simulink model "test_sim"  (R2024b)
settings: Solver=VariableStepAuto  StartTime=0.0  StopTime=10.0  RelTol=1e-3
undefined symbols (not defined in the file): ctrl, Fw, im, incenc, Lm, Lr, Ls, p, par, Rr
libraries: simulink x2
settings Model: Creator=overflow  LastModifiedBy=overflow

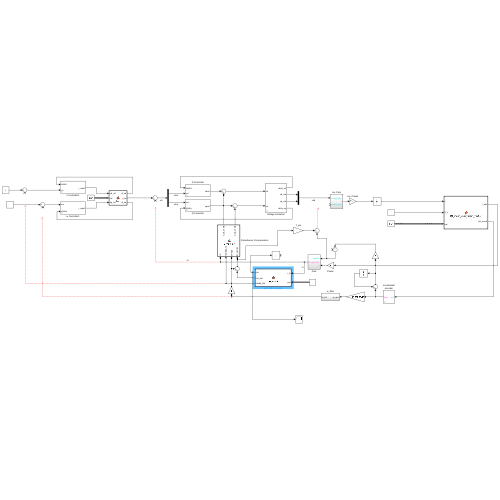
[thumbnail: Simulink's stored preview of the top-level diagram]
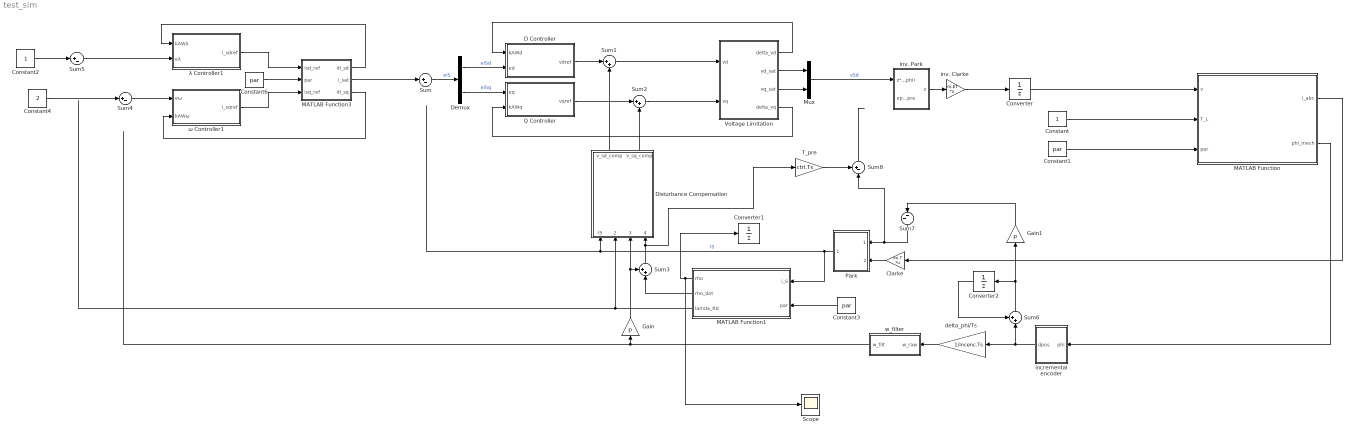
== system test_sim ==
  Clarke : Gain  Gain=im.T  Multiplication=Matrix(K*u)
  Constant : Constant
  Constant1 : Constant  Value=par  OutDataTypeStr=Bus: slBus1
  Constant2 : Constant
  Constant3 : Constant  Value=par  OutDataTypeStr=Bus: slBus1
  Constant4 : Constant  Value=2
  Constant6 : Constant  Value=par  OutDataTypeStr=Bus: slBus1
  Converter : UnitDelay  SampleTime=-1  HasFrameUpgradeWarning=on
  Converter1 : UnitDelay  SampleTime=-1  HasFrameUpgradeWarning=on
  Converter2 : UnitDelay  SampleTime=-1  HasFrameUpgradeWarning=on
  D Controller : Subsystem  mask{Ts=ctrl.Ts, ctrl=ctrl.i}
      mask prompts: Ts "Sampling Time"; ctrl "Controller Struct"
  Demux : Demux  Outputs=2
  Disturbance Compensation : MATLAB Function  TreatAsAtomicUnit=on
  Gain : Gain  Gain=p
  Gain1 : Gain  Gain=p
  MATLAB Function : MATLAB Function  TreatAsAtomicUnit=on
  MATLAB Function1 : MATLAB Function  TreatAsAtomicUnit=on
  MATLAB Function3 : MATLAB Function  TreatAsAtomicUnit=on
  Mux : Mux  Inputs=2
  Park : Subsystem
  Q Controller : Subsystem  mask{Ts=ctrl.Ts, ctrl=ctrl.i}
      mask prompts: Ts "Sampling Time"; ctrl "Controller Struct"
  Scope : Scope
  Sum : Sum  Inputs=|+-
  Sum1 : Sum  Inputs=|++  OutDataTypeStr=double  AccumDataTypeStr=double
  Sum2 : Sum  Inputs=|++  OutDataTypeStr=double  AccumDataTypeStr=double
  Sum3 : Sum  Inputs=++|
  Sum4 : Sum  Inputs=|+-
  Sum5 : Sum  Inputs=|+-
  Sum6 : Sum  Inputs=++|
  Sum7 : Sum  Inputs=--|
  Sum8 : Sum  Inputs=+-|
  T_pre : Gain  Gain=ctrl.Ts  SaturateOnIntegerOverflow=on  OutDataTypeStr=Inherit: Same as input  ParamDataTypeStr=Inherit: Same as input
  Voltage Limitation : Subsystem  mask{Vmax=im.vDC}
      mask prompts: Vmax "Max Voltage"
  delta_phi/Ts : Gain  Gain=1/incenc.Ts  SaturateOnIntegerOverflow=on  OutDataTypeStr=Inherit: Same as input  ParamDataTypeStr=Inherit: Same as input
  incremental encoder : Subsystem  mask{incenc=incenc}
      mask prompts: incenc "Parameterstruct"
  inv. Clarke : Gain  Gain=im.ET  Multiplication=Matrix(K*u)
  inv. Park : Subsystem
  w_filter : Subsystem
  λ Controller1 : Subsystem  mask{Ts=ctrl.Ts, ctrl=ctrl.w}
      mask prompts: Ts "Sampling Time"; ctrl "Controller Struct"
  ω Controller1 : Subsystem  mask{Ts=ctrl.Ts, ctrl=ctrl.w}
      mask prompts: Ts "Sampling Time"; ctrl "Controller Struct"
  wires:
  Demux/1 -> D Controller/2(ed)  "eiSd"
  w_filter/1(w_filt) -> Gain/1
  Sum1/1 -> Voltage Limitation/1(vd)
  Sum3/1 -> T_pre/1, Disturbance Compensation/4(dt_epsilon)
  Disturbance Compensation/1(v_sd_comp) -> Sum1/2
  Voltage Limitation/1(delta_vd) -> D Controller/1(kAWd)
  incremental encoder/1(dpos) -> Sum6/2, delta_phi/Ts/1
  Voltage Limitation/2(vd_sat) -> Mux/1
  T_pre/1 -> Sum8/1
  Voltage Limitation/4(delta_vq) -> Q Controller/2(kAWq)
  MATLAB Function/1(i_abc) -> Clarke/1
  ω Controller1/1(i_sqref) -> MATLAB Function3/3(isq_ref)
  Gain1/1 -> Sum7/2
  Constant/1 -> MATLAB Function/2(T_L)
  Sum4/1 -> ω Controller1/1(eω)
  Sum2/1 -> Voltage Limitation/2("vq ")
  Park/1(z*exp(j*phi)) -> MATLAB Function1/1(i_S), Disturbance Compensation/1(iS)  "iS"
  MATLAB Function1/1(rho) -> Scope/1, Converter1/1
  MATLAB Function1/2(rho_dot) -> Sum3/2
  Sum5/1 -> λ Controller1/2(eλ)
  Constant3/1 -> MATLAB Function1/2(par)
  MATLAB Function3/2(i_sat) -> Sum/1
  MATLAB Function3/1(di_sd) -> λ Controller1/1(kAWλ)
  MATLAB Function/2(phi_mech) -> incremental encoder/1(phi)
  inv. Clarke/1 -> Converter/1
  Constant6/1 -> MATLAB Function3/2(par)
  Demux/2 -> Q Controller/1(eq)  "eiSq"
  Sum8/1 -> ?
  MATLAB Function3/3(di_sq) -> ω Controller1/2(kAWω)
  Clarke/1 -> Park/2(z)
  Converter2/1 -> Sum6/1
  λ Controller1/1(i_sdref) -> MATLAB Function3/1(isd_ref)
  Constant1/1 -> MATLAB Function/3(par)
  MATLAB Function1/3(lamda_Rd) -> Disturbance Compensation/2(lambda_rd)
  Sum7/1 -> Sum8/2, Park/1(-epsilon)
  Sum/1 -> Demux/1  "eiS"
  Converter/1 -> MATLAB Function/1(v)
  Mux/1 -> inv. Park/1(z*exp(j*phi))  "vSd"
  Disturbance Compensation/2(v_sq_comp) -> Sum2/2
  Q Controller/1(vqref) -> Sum2/1
  inv. Park/1(z) -> inv. Clarke/1
  Gain/1 -> Sum3/1, Disturbance Compensation/3(omega)
  D Controller/1(vdref) -> Sum1/1
  Sum6/1 -> Gain1/1, Converter2/1
  Voltage Limitation/3(vq_sat) -> Mux/2
  Constant2/1 -> Sum5/1
  Constant4/1 -> Sum4/1
  delta_phi/Ts/1 -> w_filter/1(w_raw)

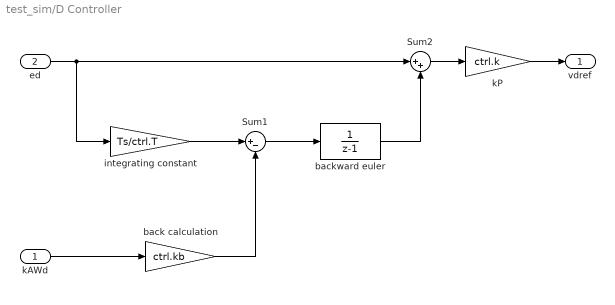
== system test_sim/D Controller ==
  kAWd : Inport
  ed : Inport  Port=2
  Sum1 : Sum  Inputs=|+-
  Sum2 : Sum  Inputs=|++
  back calculation : Gain  Gain=ctrl.kb
  backward euler : DiscreteTransferFcn  Denominator=[1 -1]
  integrating constant : Gain  Gain=Ts/ctrl.T
  kP : Gain  Gain=ctrl.k
  vdref : Outport
  wires:
  Sum1/1 -> backward euler/1
  integrating constant/1 -> Sum1/1
  back calculation/1 -> Sum1/2
  ed/1 -> integrating constant/1, Sum2/1
  Sum2/1 -> kP/1
  kP/1 -> vdref/1
  backward euler/1 -> Sum2/2
  kAWd/1 -> back calculation/1

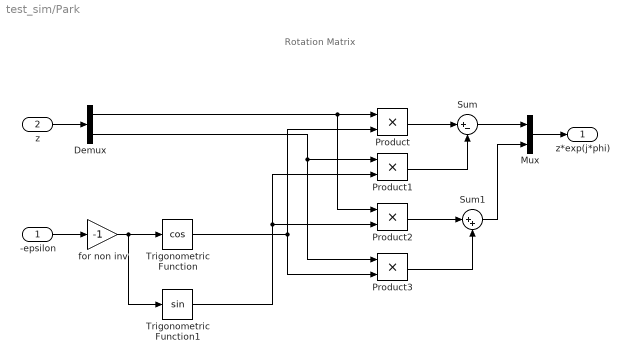
== system test_sim/Park ==
  note: Rotation Matrix
  -epsilon : Inport
  z : Inport  Port=2
  Demux : Demux  Outputs=2
      settings: DisplayOption=none
  Mux : Mux  Inputs=2
  Product{,1..3} (4 alike) : Product  SaturateOnIntegerOverflow=on  OutDataTypeStr=Inherit: Same as first input
  Sum : Sum  Inputs=|+-  SaturateOnIntegerOverflow=on
  Sum1 : Sum  Inputs=|++  SaturateOnIntegerOverflow=on
  Trigonometric Function : Trigonometry  Operator=cos
  Trigonometric Function1 : Trigonometry
  for non inv : Gain  Gain=-1
  z*exp(j*phi) : Outport  PortDimensions=2  VectorParamsAs1DForOutWhenUnconnected=off
  wires:
  Mux/1 -> z*exp(j*phi)/1
  Sum1/1 -> Mux/2
  Sum/1 -> Mux/1
  Product3/1 -> Sum1/2
  Product2/1 -> Sum1/1
  Product1/1 -> Sum/2
  Product/1 -> Sum/1
  Trigonometric Function1/1 -> Product2/2, Product1/2
  Trigonometric Function/1 -> Product3/2, Product/2
  Demux/2 -> Product3/1, Product1/1
  Demux/1 -> Product2/1, Product/1
  z/1 -> Demux/1
  -epsilon/1 -> for non inv/1
  for non inv/1 -> Trigonometric Function1/1, Trigonometric Function/1

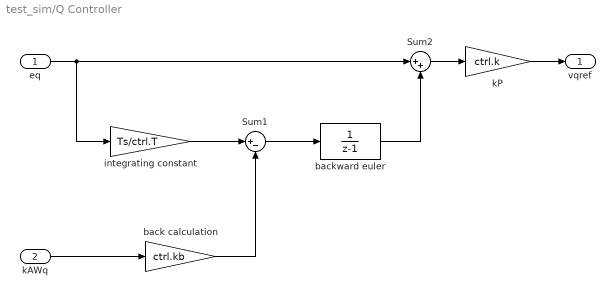
== system test_sim/Q Controller ==
  eq : Inport
  kAWq : Inport  Port=2
  Sum1 : Sum  Inputs=|+-
  Sum2 : Sum  Inputs=|++
  back calculation : Gain  Gain=ctrl.kb
  backward euler : DiscreteTransferFcn  Denominator=[1 -1]
  integrating constant : Gain  Gain=Ts/ctrl.T
  kP : Gain  Gain=ctrl.k
  vqref : Outport
  wires:
  Sum1/1 -> backward euler/1
  integrating constant/1 -> Sum1/1
  back calculation/1 -> Sum1/2
  eq/1 -> integrating constant/1, Sum2/1
  Sum2/1 -> kP/1
  kP/1 -> vqref/1
  backward euler/1 -> Sum2/2
  kAWq/1 -> back calculation/1

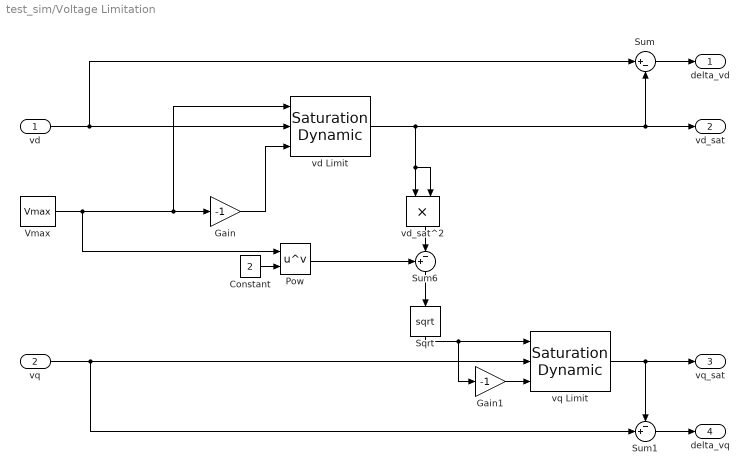
== system test_sim/Voltage Limitation ==
  vd : Inport
  "vq " : Inport  Port=2
  Constant : Constant  Value=2
  Gain : Gain  Gain=-1
  Gain1 : Gain  Gain=-1
  Pow : Math  Operator=pow  RndMeth=Zero
  Sqrt : Sqrt
  Sum : Sum  Inputs=|+-
  Sum1 : Sum  Inputs=-+|
  Sum6 : Sum  Inputs=+-|
  Vmax : Constant  Value=Vmax
  vd Limit : simulink/Discontinuities/Saturation Dynamic  OutMin=[]  OutMax=[]  OutDataTypeStr=Inherit: Same as second input  OutDataType=fixdt(1, 16)  OutScaling=2^-10  DoSatur=off
  vd_sat^2 : Product
  vq Limit : simulink/Discontinuities/Saturation Dynamic  OutMin=[]  OutMax=[]  OutDataTypeStr=Inherit: Same as second input  OutDataType=fixdt(1, 16)  OutScaling=2^-10  DoSatur=off
  delta_vd : Outport  VectorParamsAs1DForOutWhenUnconnected=off
  vd_sat : Outport  Port=2  VectorParamsAs1DForOutWhenUnconnected=off
  vq_sat : Outport  Port=3  VectorParamsAs1DForOutWhenUnconnected=off
  delta_vq : Outport  Port=4  VectorParamsAs1DForOutWhenUnconnected=off
  wires:
  Gain/1 -> vd Limit/3
  vd Limit/1 -> Sum/2, vd_sat/1, vd_sat^2/2, vd_sat^2/1
  Sqrt/1 -> Gain1/1, vq Limit/1
  vq Limit/1 -> Sum1/1, vq_sat/1
  Pow/1 -> Sum6/1
  vd/1 -> Sum/1, vd Limit/2
  Sum6/1 -> Sqrt/1
  "vq "/1 -> vq Limit/2, Sum1/2
  vd_sat^2/1 -> Sum6/2
  Vmax/1 -> Pow/1, Gain/1, vd Limit/1
  Gain1/1 -> vq Limit/3
  Sum/1 -> delta_vd/1
  Sum1/1 -> delta_vq/1
  Constant/1 -> Pow/2

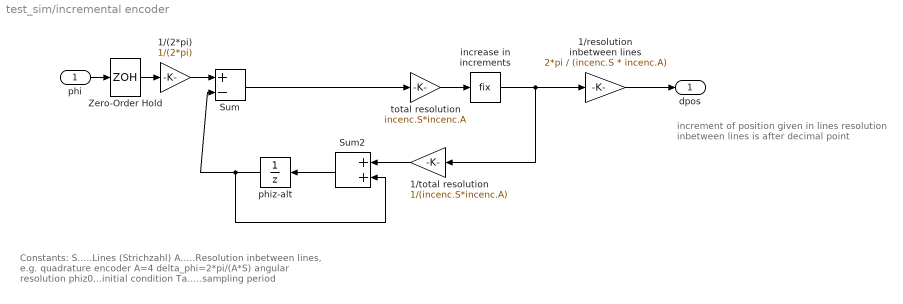
== system test_sim/incremental encoder ==
  note: increment of position given in lines
      | resolution inbetween lines is after decimal point
  note: Constants:
      | S.....Lines (Strichzahl)
      | A.....Resolution inbetween lines, e.g. quadrature encoder A=4
      |        delta_phi=2*pi/(A*S) angular resolution
      | phiz0...initial condition
      | Ta.....sampling period
  phi : Inport
  1/(2*pi) : Gain  Gain=1/(2*pi)  OutDataTypeStr=Inherit: Same as input  ParamDataTypeStr=Inherit: Same as input
  1/resolution inbetween lines : Gain  Gain=2*pi / (incenc.S * incenc.A)  OutDataTypeStr=Inherit: Same as input  ParamDataTypeStr=Inherit: Same as input
  1/total resolution : Gain  Gain=1/(incenc.S*incenc.A)  OutDataTypeStr=Inherit: Same as input  ParamDataTypeStr=Inherit: Same as input
  Sum : Sum  Inputs=+-  InputSameDT=on  OutDataTypeStr=Inherit: Same as first input
  Sum2 : Sum  InputSameDT=on  OutDataTypeStr=Inherit: Same as first input
  Zero-Order Hold : ZeroOrderHold  SampleTime=incenc.Ts
  increase in increments : Rounding  Operator=fix
  phiz-alt : UnitDelay  InitialCondition=incenc.phiz0  SampleTime=incenc.Ts  HasFrameUpgradeWarning=on
  total resolution : Gain  Gain=incenc.S*incenc.A  OutDataTypeStr=Inherit: Same as input  ParamDataTypeStr=Inherit: Same as input
  dpos : Outport  VectorParamsAs1DForOutWhenUnconnected=off
  wires:
  Sum2/1 -> phiz-alt/1
  1/total resolution/1 -> Sum2/1
  1/(2*pi)/1 -> Sum/1
  increase in increments/1 -> 1/resolution inbetween lines/1, 1/total resolution/1
  phi/1 -> Zero-Order Hold/1
  phiz-alt/1 -> Sum2/2, Sum/2
  total resolution/1 -> increase in increments/1
  Sum/1 -> total resolution/1
  Zero-Order Hold/1 -> 1/(2*pi)/1
  1/resolution inbetween lines/1 -> dpos/1

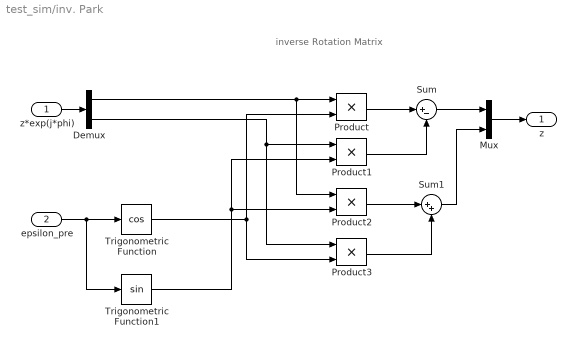
== system test_sim/inv. Park ==
  note: inverse Rotation Matrix
  z*exp(j*phi) : Inport
  epsilon_pre : Inport  Port=2
  Demux : Demux  Outputs=2
      settings: DisplayOption=none
  Mux : Mux  Inputs=2
  Product{,1..3} (4 alike) : Product  SaturateOnIntegerOverflow=on  OutDataTypeStr=Inherit: Same as first input
  Sum : Sum  Inputs=|+-  SaturateOnIntegerOverflow=on
  Sum1 : Sum  Inputs=|++  SaturateOnIntegerOverflow=on
  Trigonometric Function : Trigonometry  Operator=cos
  Trigonometric Function1 : Trigonometry
  z : Outport  PortDimensions=2  VectorParamsAs1DForOutWhenUnconnected=off
  wires:
  z*exp(j*phi)/1 -> Demux/1
  Demux/1 -> Product/1, Product2/1
  epsilon_pre/1 -> Trigonometric Function1/1, Trigonometric Function/1
  Demux/2 -> Product1/1, Product3/1
  Trigonometric Function/1 -> Product/2, Product3/2
  Trigonometric Function1/1 -> Product1/2, Product2/2
  Product/1 -> Sum/1
  Product1/1 -> Sum/2
  Product2/1 -> Sum1/1
  Product3/1 -> Sum1/2
  Sum/1 -> Mux/1
  Sum1/1 -> Mux/2
  Mux/1 -> z/1

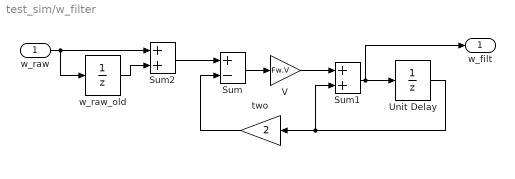
== system test_sim/w_filter ==
  w_raw : Inport
  Sum : Sum  Inputs=+-  SaturateOnIntegerOverflow=on
  Sum1 : Sum  SaturateOnIntegerOverflow=on
  Sum2 : Sum  SaturateOnIntegerOverflow=on
  Unit Delay : UnitDelay  InitialCondition=Fw.w0  SampleTime=Fw.Ts  HasFrameUpgradeWarning=on
  V : Gain  Gain=Fw.V  SaturateOnIntegerOverflow=on  OutDataTypeStr=Inherit: Same as input  ParamDataTypeStr=Inherit: Same as input
  two : Gain  Gain=2  SaturateOnIntegerOverflow=on  OutDataTypeStr=Inherit: Same as input  ParamDataTypeStr=Inherit: Same as input
  w_raw_old : UnitDelay  InitialCondition=Fw.w0  SampleTime=Fw.Ts  HasFrameUpgradeWarning=on
  w_filt : Outport  VectorParamsAs1DForOutWhenUnconnected=off
  wires:
  Sum1/1 -> Unit Delay/1, w_filt/1
  Sum/1 -> V/1
  Sum2/1 -> Sum/1
  V/1 -> Sum1/1
  two/1 -> Sum/2
  Unit Delay/1 -> two/1, Sum1/2
  w_raw_old/1 -> Sum2/2
  w_raw/1 -> w_raw_old/1, Sum2/1

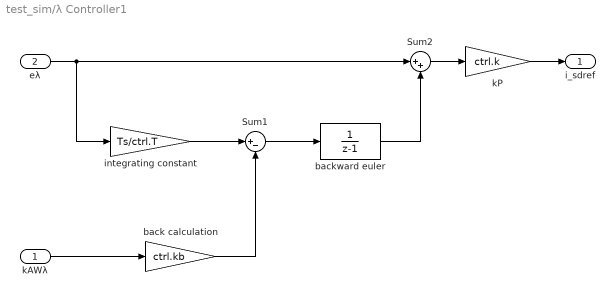
== system test_sim/λ Controller1 ==
  kAWλ : Inport
  eλ : Inport  Port=2
  Sum1 : Sum  Inputs=|+-
  Sum2 : Sum  Inputs=|++
  back calculation : Gain  Gain=ctrl.kb
  backward euler : DiscreteTransferFcn  Denominator=[1 -1]
  integrating constant : Gain  Gain=Ts/ctrl.T
  kP : Gain  Gain=ctrl.k
  i_sdref : Outport
  wires:
  Sum1/1 -> backward euler/1
  integrating constant/1 -> Sum1/1
  back calculation/1 -> Sum1/2
  eλ/1 -> integrating constant/1, Sum2/1
  Sum2/1 -> kP/1
  kP/1 -> i_sdref/1
  backward euler/1 -> Sum2/2
  kAWλ/1 -> back calculation/1

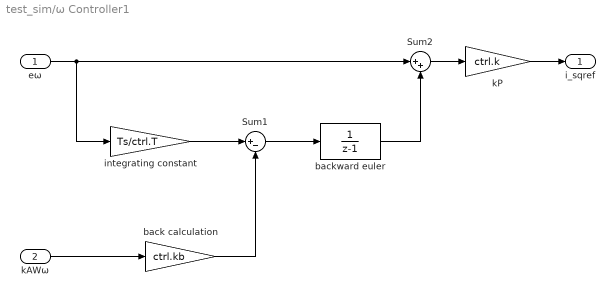
== system test_sim/ω Controller1 ==
  eω : Inport
  kAWω : Inport  Port=2
  Sum1 : Sum  Inputs=|+-
  Sum2 : Sum  Inputs=|++
  back calculation : Gain  Gain=ctrl.kb
  backward euler : DiscreteTransferFcn  Denominator=[1 -1]
  integrating constant : Gain  Gain=Ts/ctrl.T
  kP : Gain  Gain=ctrl.k
  i_sqref : Outport
  wires:
  Sum1/1 -> backward euler/1
  integrating constant/1 -> Sum1/1
  back calculation/1 -> Sum1/2
  eω/1 -> integrating constant/1, Sum2/1
  Sum2/1 -> kP/1
  kP/1 -> i_sqref/1
  backward euler/1 -> Sum2/2
  kAWω/1 -> back calculation/1

== matlab function test_sim/MATLAB Function1 ==
  data: rho output; rho_dot output; i_S input; lamda_Rd output; par input
function [rho, rho_dot, lamda_Rd] = flux_model(i_S, par)

i_sd = i_S(1);
i_sq = i_S(2);

% PARAMETERS
Ts = par.Ts;
p  = par.p;
Jm = par.J;

Rs = par.Rs;
Rr = par.Rr;

Ls = par.Ls;     % LσS
Lr = par.Lr;     % L'σR
Lm  = par.Lm;

Tau_R = Lr/Rr;

persistent rho_k lamda_Rd_k
if isempty(rho_k) 
    rho_k = 0;
    lamda_Rd_k = 0.01;
end

lamda_Rd_k = lamda_Rd_k + Ts / Tau_R * (Lm * i_sd - lamda_Rd_k);

rho_dot = Lm * i_sq / (Tau_R * lamda_Rd_k);

rho_k = rho_k + Ts * rho_dot;

lamda_Rd = lamda_Rd_k;
rho = rho_k;

== matlab function test_sim/Disturbance Compensation ==
  data: iS input; v_sd_comp output; lambda_rd input; omega input; dt_epsilon input; Ls parameter; Lm parameter; Lr parameter; Rr parameter; v_sq_comp output
function [v_sd_comp, v_sq_comp]  = Decoupling(iS, lambda_rd, omega, dt_epsilon, Ls, Lm, Lr, Rr)

i_Sd = iS(1);
i_Sq = iS(2);



% convenience;  (3.15) unter satz
L_sigma=(Ls - Lm^2/Lr); 

% compensation
% v_sd_comp = -dt_epsilon*L_sigma*i_Sq - Rr *  Lm/Lr^2 * lambda_rd;  % (3.21)
% v_sq_comp =  dt_epsilon*L_sigma*i_Sd + omega * Lm/Lr^2 * lambda_rd; % (3.22)

v_sd_comp = 0.0;
v_sq_comp = 0.0;

== matlab function test_sim/MATLAB Function ==
  data: v input; i_abc output; T_L input; phi_mech output; par input
function [i_abc, phi_mech] = IM_mech_subsystem_vector(v,T_L,par)

va = v(1);
vb = v(2);
vc = v(3);

% Vector formulation consistent with IM_Model (Seebacher)
% States: lambdaS (stator flux), lambdaR (rotor flux, referred), omega_mech

% PARAMETERS
Ts = par.Ts;
p  = par.p;
Jm = par.J;

Rs = par.Rs;
Rr = par.Rr;

Ls = par.Ls;     
Lr = par.Lr;     
Lm  = par.Lm;

B = 0;

% CONSTANT MATRICES
J = [0 -1; 1 0];   % 90° rotation matrix

T_abc_albe = (2/3)*[ 1  -1/2  -1/2;
                     0  sqrt(3)/2 -sqrt(3)/2 ];

T_albe_abc = [ 1   0;
              -1/2  sqrt(3)/2;
              -1/2 -sqrt(3)/2 ];

% STATES
persistent lambdaS lambdaR omega_k phi_k
if isempty(lambdaS)
    lambdaS = zeros(2,1);   % λ_S
    lambdaR = zeros(2,1);   % λ'_R
    omega_k = 0;            % ω_mech
    phi_k = 0;
end

% INPUT TRANSFORMATION
vS = T_abc_albe*[va;vb;vc];   % v_S (αβ)

% ELECTRICAL SPEED
omega = p*omega_k;            % ω = p·ω_mech

% CURRENT CALCULATION (consistent with 6.9 / 6.10)
% lambdaS = Lls*iS + lambda_m
% lambdaR = Llr*iR + lambda_m
% lambda_m = Lm*(iS + iR)

% Solve for lambda_m first:
den = 1 + Lm*(1/Ls + 1/Lr);
lambda_m = (Lm/den) * ( (1/Ls)*lambdaS + (1/Lr)*lambdaR );

% Then currents:
iS = (lambdaS - lambda_m)/Ls;
iR = (lambdaR - lambda_m)/Lr;

% FLUX DERIVATIVES (6.8 / 6.6)
dlambdaS = vS - Rs*iS;
dlambdaR = -Rr*iR + omega*J*lambdaR;

% ELECTROMAGNETIC TORQUE (use lambda_m, not lambdaS)
Te = (3/2)*p*(lambda_m.'*J*iS);

% MECHANICS
domega = (Te - T_L - B*omega_k)/Jm;

% INTEGRATION (Euler)
lambdaS = lambdaS + Ts*dlambdaS;
lambdaR = lambdaR + Ts*dlambdaR;
omega_k = omega_k + Ts*domega;

phi_k = phi_k + Ts*omega;

phi_mech = phi_k;

% OUTPUT CURRENTS abc
i_abc = T_albe_abc*iS;

end

== matlab function test_sim/MATLAB Function3 ==
  data: isd_ref input; par input; di_sd output; isq_ref input; i_sat output; di_sq output
function [di_sd, i_sat, di_sq] = fcn(isd_ref, par, isq_ref)

isd_max = par.k_is * par.is_max;

isd_sat = max([min(isd_ref, isd_max), -isd_max]);

di_sd = isd_ref - isd_sat;

isq_max = sqrt(par.is_max^2 -  isd_sat^2);

isq_sat = max([min(isq_ref, isq_max), -isq_max]);

di_sq = isq_ref - isq_sat;

i_sat = [isd_sat, isq_sat];
